simulink model "MSE483Project_StateSpaceForm"  (R2020b)
settings: Solver=ode15s  StartTime=0.0  StopTime=50  MaxStep=1e-5  RelTol=1e-3
InitFcn:
  | A=[0,  0,           1,          0;
  |     0,  0,           0,          1;
  |     0, -409.7184,  -104.6299,   104.6299;
  |     0,  268.6273,    54.5833,   -54.5833]
  | B = [0;0;101.6952;-53.0523]
  | C=[1 0 0 0]
  | D=[0]
  | x0=[0;90*pi/180;0;0]
  | K=[-318.517516293979	-839.316963783976	-66.2263834004483	-127.491021126397]
  | KI = 890.808276084874
  | Ob= [ 400.0000   ,      0   , 1.0000  , 0;
  |          0 , 400.0000   ,      0  ,  1.0000;
  |          0, -409.718, 295.3701 , 104.6299;
  |          0,  268.6273 ,  54.5833 , 345.4167]
settings Model: Creator=samuel  LastModifiedBy=mkupp

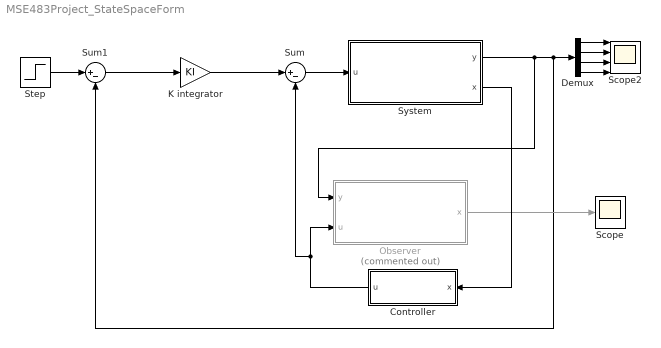
== system MSE483Project_StateSpaceForm ==
  Controller : Subsystem
  Demux : Demux
  K integrator : Gain  InitFcn=|  Gain=KI
      | A=[0,  0,           1,          0;
      |     0,  0,           0,          1;
      |     0, -409.7184,  -104.6299,   104.6299;
      |     0,  268.6273,    54.5833,   -54.5833]
      | B = [0;0;101.6952;-53.0523]
      | C=[1 0 0 0]
      | D=[0]
      | x0=[0;90*pi/180;0;0]
      | K=[-62.8966122663488	-201.905572339641	-14.9133345772124	-27.6218237282572]
      | Ob= [ 400.0000   ,      0   , 1.0000  ,       0;
      |          0 , 400.0000   ,      0  ,  1.0000;
      |          0, -409.718, 295.3701 , 104.6299;
      |          0,  268.6273 ,  54.5833 , 345.4167]
  Observer : Subsystem  Commented=on
  Scope : Scope
  Scope2 : Scope  NumInputPorts=4
  Step : Step  SampleTime=0
  Sum : Sum  Inputs=|+-
  Sum1 : Sum  Inputs=|+-
  System : Subsystem
  wires:
  Sum/1 -> System/1(u)
  Controller/1(u) -> Sum/2, Observer/2(u)
  System/1(y) -> Sum1/2, Demux/1, Observer/1(y)
  Observer/1(x) -> Scope/1
  System/2(x) -> Controller/1(x)
  Demux/1 -> Scope2/1
  Demux/2 -> Scope2/2
  Demux/3 -> Scope2/3
  Demux/4 -> Scope2/4
  K integrator/1 -> Sum/1
  Step/1 -> Sum1/1
  Sum1/1 -> K integrator/1

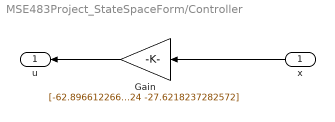
== system MSE483Project_StateSpaceForm/Controller ==
  x : Inport
  Gain : Gain  Gain="[-62.8966122663488 -201.905572339641\t-14.9133345772124\t-27.6218237282572]"
  u : Outport
  wires:
  Gain/1 -> u/1
  x/1 -> Gain/1

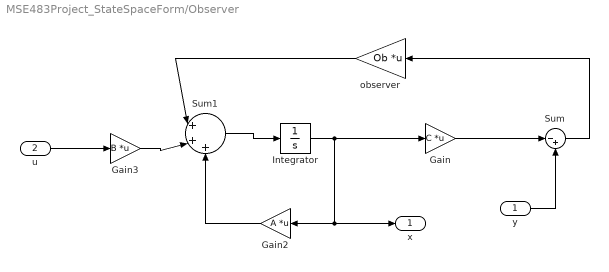
== system MSE483Project_StateSpaceForm/Observer ==
  y : Inport
  u : Inport  Port=2
  Gain : Gain  Gain=C  Multiplication=Matrix(K*u)
  Gain2 : Gain  Gain=A  Multiplication=Matrix(K*u)
  Gain3 : Gain  Gain=B  Multiplication=Matrix(K*u)
  Integrator : Integrator  InitialCondition=x0
  Sum : Sum  Inputs=|-+
  Sum1 : Sum  Inputs=|+++
  observer : Gain  Gain=Ob  Multiplication=Matrix(K*u)
  x : Outport
  wires:
  u/1 -> Gain3/1
  Gain/1 -> Sum/1
  Sum1/1 -> Integrator/1
  Integrator/1 -> Gain2/1, x/1, Gain/1
  y/1 -> Sum/2
  Sum/1 -> observer/1
  observer/1 -> Sum1/1
  Gain3/1 -> Sum1/2
  Gain2/1 -> Sum1/3

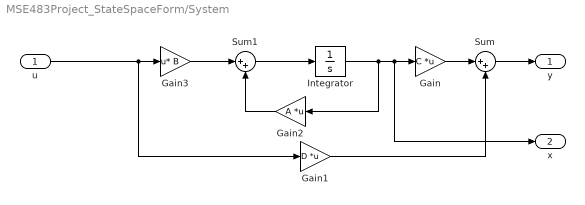
== system MSE483Project_StateSpaceForm/System ==
  u : Inport
  Gain : Gain  Gain=C  Multiplication=Matrix(K*u)
  Gain1 : Gain  Gain=D  Multiplication=Matrix(K*u)
  Gain2 : Gain  Gain=A  Multiplication=Matrix(K*u)
  Gain3 : Gain  Gain=B  Multiplication=Matrix(u*K)
  Integrator : Integrator  InitialCondition=x0
  Sum : Sum  Inputs=|++
  Sum1 : Sum  Inputs=|++
  y : Outport
  x : Outport  Port=2
  wires:
  Integrator/1 -> Gain2/1, x/1, Gain/1
  u/1 -> Gain1/1, Gain3/1
  Gain/1 -> Sum/1
  Sum1/1 -> Integrator/1
  Gain2/1 -> Sum1/2
  Gain3/1 -> Sum1/1
  Gain1/1 -> Sum/2
  Sum/1 -> y/1
